simulink library "dlbsBlockSin"  (R2025b)
settings: Solver=VariableStepAuto  StartTime=0.0  StopTime=10.0  RelTol=1e-3
libraries: dlbsBlockExtractGradientGF x1, dlbsBlockInsertGradientGF x1
settings Model: Creator=lt6037  LastModifiedBy=lt6037

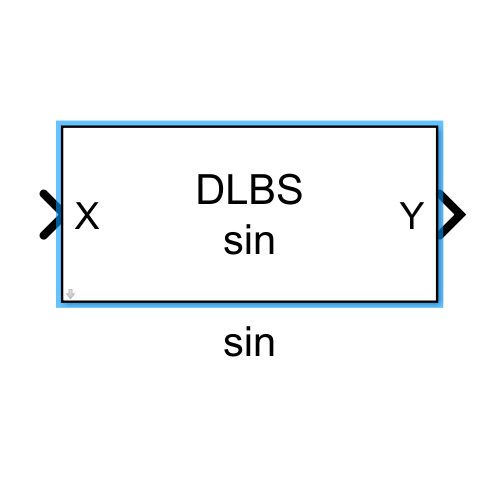
[thumbnail: Simulink's stored preview of the top-level diagram]
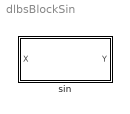
== system dlbsBlockSin ==
  sin : Subsystem
      mask help: Applies the sine function to the input tensor. The operation is applied element-wise across all tensor elements.
      mask Help: web("dlbsHelpBlockSin.html")
      mask Display: fprintf("DLBS\nsin");

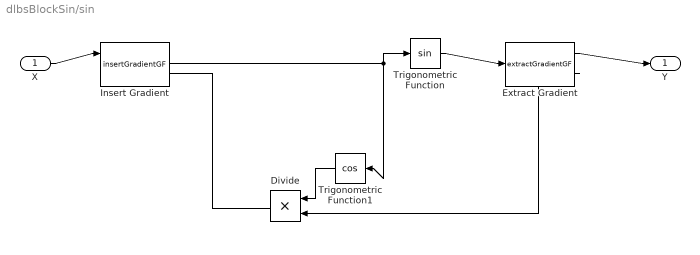
== system dlbsBlockSin/sin ==
  X : Inport
  Divide : Product  Inputs=**
  Extract Gradient : dlbsBlockExtractGradientGF/extractGradientGF
  Insert Gradient : dlbsBlockInsertGradientGF/insertGradientGF
  Trigonometric Function : Trigonometry
  Trigonometric Function1 : Trigonometry  Operator=cos
  Y : Outport
  wires:
  Insert Gradient/1 -> Trigonometric Function1/1, Trigonometric Function/1
  Divide/1 -> Insert Gradient/2
  Trigonometric Function/1 -> Extract Gradient/1
  Extract Gradient/1 -> Y/1
  X/1 -> Insert Gradient/1
  Trigonometric Function1/1 -> Divide/1
  Extract Gradient/2 -> Divide/2
